simulink model "xebamline"  (R2018a)
settings: Solver=ode5  StartTime=0.0  StopTime=120  FixedStep=0.1  RelTol=1e-3
undefined symbols (not defined in the file): sigbuilder_block
libraries: fuzblock x1
settings Model: Creator=DELL  LastModifiedBy=DELL

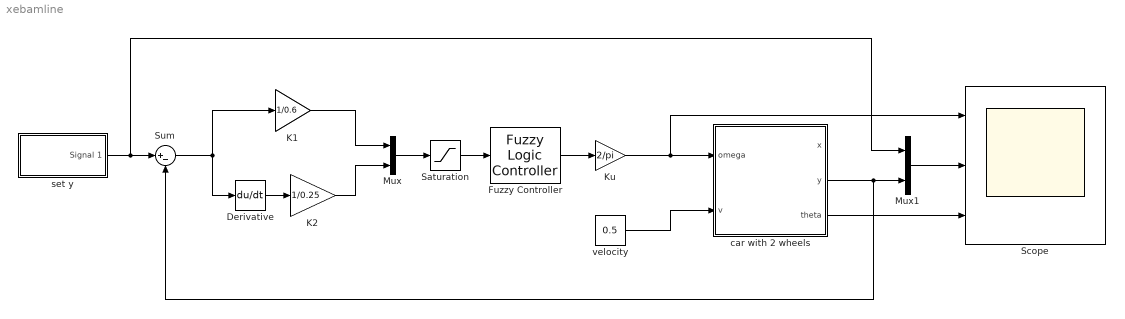
== system xebamline ==
  Derivative : Derivative
  Fuzzy Controller : fuzblock/Fuzzy Logic  Controller  FIS='fuzzy1.fis'  OutputSampleNumber=101  DataType=double  FuzzifiedInputs=off  RuleFiringStrengths=off  RuleOutputs=off  AggregatedOutputs=off  SimulateUsing=Interpreted execution  OutOfRangeInputValueMessage=warning  NoRuleFiredMessage=warning  EmptyOutputFuzzySetMessage=warning
  K1 : Gain  Gain=1/0.6
  K2 : Gain  Gain=1/0.25
  Ku : Gain  Gain=2/pi
  Mux : Mux  Inputs=2
  Mux1 : Mux  Inputs=2
  Saturation : Saturate  UpperLimit=1  LowerLimit=-1
  Scope : Scope  NumInputPorts=3
  Sum : Sum  Inputs=|+-
  car with 2 wheels : Subsystem
  set y : Subsystem  Tag=STV Subsys  LoadFcn=sigbuilder_block('load');  StartFcn=sigbuilder_block('start');  StopFcn=sigbuilder_block('stop');  ClipboardFcn=sigbuilder_block('clipboard');  mask(Sigbuilder block){tuvar=[0:10]}
      mask help: Simulink:masks:SigbuilderBlock_MD
      mask init:
      | if ~strcmp(get_param(bdroot(gcbh),'SimulationStatus'),'stopped') tuvar = sigbuilder_block('maskInit'); end
      settings: CopyFcn=sigbuilder_block('copy');  DeleteFcn=sigbuilder_block('delete');  ModelCloseFcn=sigbuilder_block('modelClose');  PreSaveFcn=sigbuilder_block('preSave');  PauseFcn=sigbuilder_block('pause');  ContinueFcn=sigbuilder_block('continue');  NameChangeFcn=sigbuilder_block('namechange');  OpenFcn=sigbuilder_block('open',[5.4 30 1141.2 522.6 ]);  CloseFcn=sigbuilder_block('close');
      mask Display: plot(0, 0, 100, 100,[2, 2, 32, 32, 2], [68, 8, 8, 68, 68],[32, 2], [38, 38], [32, 19, 2],[53, 60, 44], [32, 17, 17, 2],[16, 16, 31, 31]);txt = getActiveGroup(gcbh);text(2, 100, txt,'verticalAlignment', 'top');
  velocity : Constant  Value=0.5
  wires:
  Fuzzy Controller/1 -> Ku/1
  velocity/1 -> car with 2 wheels/2(v)
  Mux/1 -> Saturation/1
  K1/1 -> Mux/1
  K2/1 -> Mux/2
  car with 2 wheels/2(y) -> Mux1/2, Sum/2
  Sum/1 -> K1/1, Derivative/1
  Derivative/1 -> K2/1
  Ku/1 -> car with 2 wheels/1(omega), Scope/1
  set y/1(Signal 1) -> Sum/1, Mux1/1
  Saturation/1 -> Fuzzy Controller/1
  Mux1/1 -> Scope/2
  car with 2 wheels/3(theta) -> Scope/3

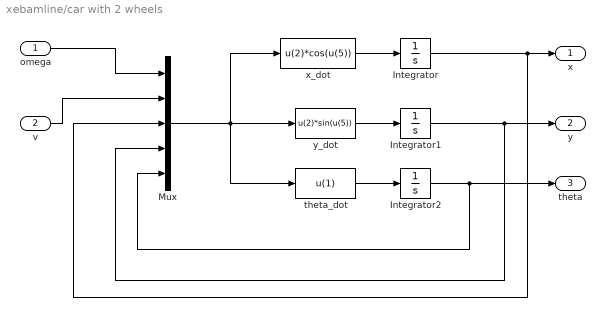
== system xebamline/car with 2 wheels ==
  omega : Inport
  v : Inport  Port=2
  Integrator : Integrator
  Integrator1 : Integrator
  Integrator2 : Integrator
  Mux : Mux  Inputs=5
  theta_dot : Fcn  Expr=u(1)
  x_dot : Fcn  Expr=u(2)*cos(u(5))
  y_dot : Fcn  Expr=u(2)*sin(u(5))
  x : Outport
  y : Outport  Port=2
  theta : Outport  Port=3
  wires:
  x_dot/1 -> Integrator/1
  Integrator/1 -> Mux/3, x/1
  theta_dot/1 -> Integrator2/1
  Integrator2/1 -> Mux/5, theta/1
  y_dot/1 -> Integrator1/1
  Integrator1/1 -> Mux/4, y/1
  omega/1 -> Mux/1
  v/1 -> Mux/2
  Mux/1 -> theta_dot/1, x_dot/1, y_dot/1

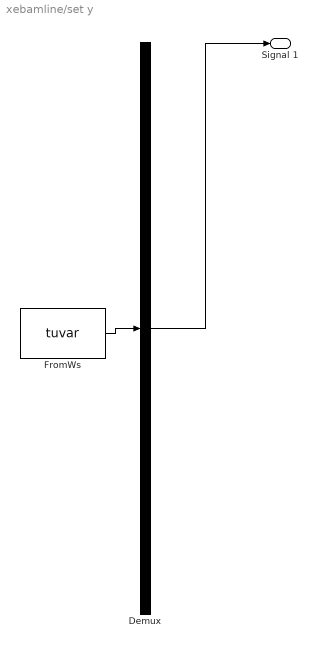
== system xebamline/set y ==
  Demux : Demux  Tag=STV Demux  Outputs=1
  FromWs : FromWorkspace  Tag=STV FromWs  VariableName=tuvar  SampleTime=0
      SigBuilderData=|
      | common.afterFinalStr = 'Extrapolate'
      | common.sampleTime = 0
      | dataSet.timeRange = [0 120]
      | dataSet.name = 'Group 1'
      | sbobj.Groups.Name = 'Group 1'
      | sbobj.Groups.Signals.Name = 'Signal 1'
      | sbobj.Groups.Signals.XData = [0 30.5 30.5 59.9 59.9 90.2 90.2 120]
      | sbobj.Groups.Signals.YData = [0.304 0.304 0.1 0.1 0.572 0.572 0.4 0.4]
      | sbobj.Groups.TimeRange = [0 120]
  Signal 1 : Outport  Tag=STV Outport
  wires:
  Demux/1 -> Signal 1/1
  FromWs/1 -> Demux/1
